simulink model "PeopleDetection_HD"  (R2020a)
settings: Solver=VariableStepAuto  StartTime=0.0  StopTime=10.0  RelTol=1e-3
settings Model: Creator=HannesDittmann  LastModifiedBy=HannesDittmann

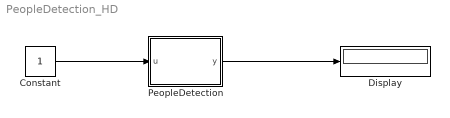
== system PeopleDetection_HD ==
  Constant : Constant
  Display : Display
  PeopleDetection : MATLAB Function  TreatAsAtomicUnit=on
  wires:
  Constant/1 -> PeopleDetection/1(u)
  PeopleDetection/1(y) -> Display/1

== matlab function PeopleDetection_HD/PeopleDetection ==
  data: u input; y output
function y = fcn(u)

y = u;
